simulink model "selector_port_2"  (R2017b)
settings: Solver=FixedStepAuto  StartTime=0.0  StopTime=0  FixedStep=0.1  MaxStep=1  RelTol=1e-3  EnableMultiTasking=on
model workspace (MAT data in the model file):
  compositionalMap.analysisNames = {'selector_port_2_PP/Selector'}
  compositionalMap.compositionalOptions = {{''}}
  compositionalMap.selectedOptions = 1
  nodeNameToBlockNameMap : containers.Map (value not decoded)
  verificationResults.analysisResults{1}.top = 'selector_port_2_PP/Selector'
  verificationResults.analysisResults{1}.abstract = ''
  verificationResults.analysisResults{1}.concrete = 'real_to_int,_Floor,_Ceiling'
  verificationResults.analysisResults{1}.assumptions = ''
  verificationResults.analysisResults{1}.properties{1}.propertyName = 'Selector_2684_830_OUTOFBOUND_1'
  verificationResults.analysisResults{1}.properties{1}.answer = 'SAFE'
  verificationResults.analysisResults{1}.properties{1}.originPath = 'selector_port_2_PP/Selector'
  verificationResults.analysisResults{1}.properties{1}.propertyType = 'Out of Bound Array Access'
  verificationResults.analysisResults{1}.properties{2}.propertyName = 'Selector_2684_830_OUTOFBOUND_3'
  verificationResults.analysisResults{1}.properties{2}.answer = 'SAFE'
  verificationResults.analysisResults{1}.properties{2}.originPath = 'selector_port_2_PP/Selector'
  verificationResults.analysisResults{1}.properties{2}.propertyType = 'Out of Bound Array Access'
  verificationResults.sampleTime = 1
settings Model: Creator=arnaud  LastModifiedBy=hbourbou
settings DataIOCC: ExternalInput=xin  LimitDataPoints=on  SaveFormat=Structure  SignalLoggingSaveFormat=ModelDataLogs
settings OptimizationCC: ExpressionDepthLimit=2147483647  LifeSpan=inf
settings DebuggingCC: UnderspecifiedInitializationDetection=Classic  MergeDetectMultiDrivingBlocksExec=none  SolverPrmCheckMsg=warning  FcnCallInpInsideContextMsg=warning  StateNameClashWarn=warning  SFUnexpectedBacktrackingDiag=warning  SFNoUnconditionalDefaultTransitionDiag=warning  SFExecutionAtInitializationDiag=none
settings HardwareCC: ProdBitPerPointer=32  ProdBitPerSizeT=32  ProdBitPerPtrDiffT=32  ProdLargestAtomicFloat=None  ProdIntDivRoundTo=Undefined  ProdEndianess=Unspecified  ProdWordSize=32  ProdHWDeviceType=32-bit Generic
settings ModelReferenceCC: PropagateSignalLabelsOutOfModel=off
settings CodeAppCC: StateflowObjectComments=on
settings GRTTargetCC: TargetLangStandard=C89/C90 (ANSI)  GeneratePreprocessorConditionals=Disable all  CombineOutputUpdateFcns=off  GRTInterface=on
settings ConfigComp: CovMetricSettings=dw  CovHtmlReporting=on  CovSaveCumulativeToWorkspaceVar=on  CovSaveSingleToWorkspaceVar=on  CovExternalEMLEnable=off  CovSFcnEnable=off

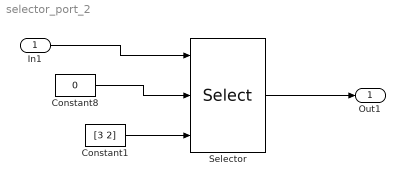
== system selector_port_2 ==
  In1 : Inport  PortDimensions=[4, 4, 4, 4]
  Constant1 : Constant  Value=[3 2]
  Constant8 : Constant  Value=0
  Selector : Selector  NumberOfDimensions=4  IndexMode=Zero-based  InputPortWidth=3  IndexOptions=Starting index (port),Starting index (dialog),Index vector (port),Select all  Indices=[1 0 0],2,1,1  OutputSizes=2,1,1,1
  Out1 : Outport
  wires:
  Selector/1 -> Out1/1
  Constant8/1 -> Selector/2
  In1/1 -> Selector/1
  Constant1/1 -> Selector/3
